simulink model "PMSM_control"  (R2021a)
settings: Solver=ode4  StartTime=0.0  StopTime=1  FixedStep=1e-5  RelTol=1e-3
libraries: spsMosfetLib x6, spsCurrentMeasurementLib x3, spsDCVoltageSourceLib x1, pid_lib x1, spsPermanentMagnetSynchronousMachineLib x1, spspowerguiLib x1
settings Model: Creator=322-PC  LastModifiedBy=juhyung
settings SolverCC: AlgebraicLoopSolver=TrustRegion
settings OptimizationCC: LifeSpan=inf
settings DebuggingCC: SFMachineParentedDataDiag=warning  ArithmeticOperatorsInVariantConditions=warning
settings SFSimCC: CustomCodeUndefinedFunction=UseInterfaceOnly
settings CodeAppCC: StateflowObjectComments=on

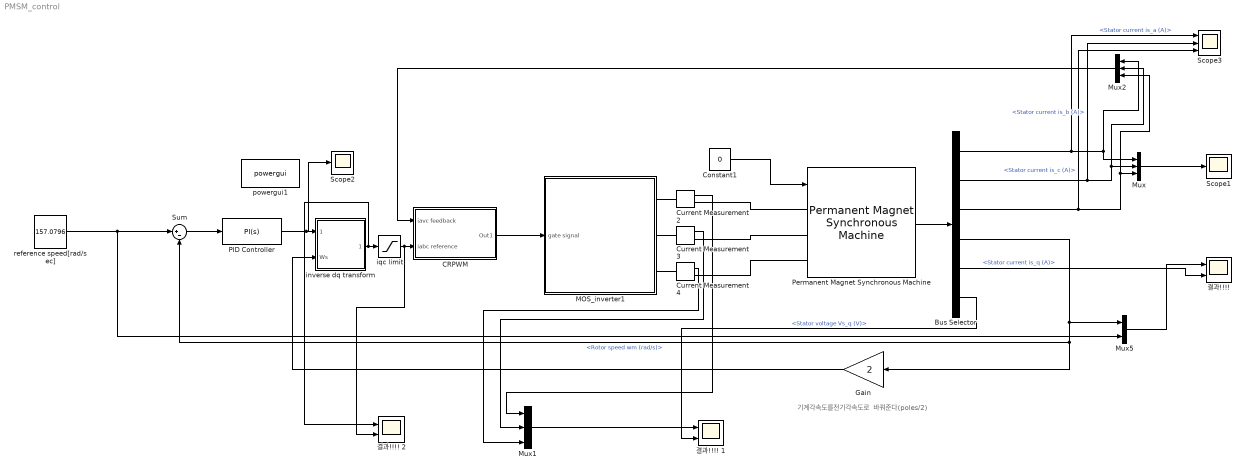
== system PMSM_control ==
  note: 기계각속도를전기각속도로 바꿔준다(poles/2)
  Bus Selector : BusSelector  OutputSignals=Stator current is_a (A),Stator current is_b (A),Stator current is_c (A),Rotor speed wm (rad/s),Stator current is_q (A),Stator voltage Vs_q (V)
  "CRPWM " : Subsystem
  Constant1 : Constant  Value=0
  Current Measurement2 : spsCurrentMeasurementLib/Current Measurement  PhasorSimulation=off  OutputType=Complex  PSBequivalent=0
  Current Measurement3 : spsCurrentMeasurementLib/Current Measurement  PhasorSimulation=off  OutputType=Complex  PSBequivalent=0
  Current Measurement4 : spsCurrentMeasurementLib/Current Measurement  PhasorSimulation=off  OutputType=Complex  PSBequivalent=0
  Gain : Gain  Gain=2
  MOS_inverter1 : Subsystem
  Mux : Mux  Inputs=3
  Mux1 : Mux  Inputs=3
  Mux2 : Mux  Inputs=3
  Mux5 : Mux  Inputs=2
  PID Controller : pid_lib/PID Controller  Controller=PI  Form=Parallel  TimeDomain=Continuous-time  UseExternalTs=off  SampleTime=-1  IntegratorMethod=Forward Euler  FilterMethod=Forward Euler  ControllerParametersSource=internal  P=0.00055  I=0.00303  D=0  UseFilter=on  N=100  TunerSelectOption=Transfer Function Based (PID Tuner App)  InitialConditionSource=internal  InitialConditionForIntegrator=0  InitialConditionForFilter=0  DifferentiatorICPrevScaledInput=0  ExternalReset=none  TrackingMode=off  Kt=1  LimitOutput=off  SatLimitsSource=internal  UpperSaturationLimit=inf  LowerSaturationLimit=-inf  LinearizeAsGain=on  AntiWindupMode=none  Kb=1  POutMin=[]  POutMax=[]  IOutMin=[]  IOutMax=[]  DOutMin=[]  DOutMax=[]  NOutMin=[]  NOutMax=[]  SumOutMin=[]  SumOutMax=[]  SaturationOutMin=[]  SaturationOutMax=[]  PParamMin=[]  PParamMax=[]  IParamMin=[]  IParamMax=[]  DParamMin=[]  DParamMax=[]  NParamMin=[]  NParamMax=[]  KbParamMin=[]  KbParamMax=[]  KtParamMin=[]  KtParamMax=[]  KbOutMin=[]  KbOutMax=[]  KtOutMin=[]  KtOutMax=[]  IntegratorOutMin=[]  IntegratorOutMax=[]  FilterOutMin=[]  FilterOutMax=[]  SumI1OutMin=[]  SumI1OutMax=[]  SumI2OutMin=[]  SumI2OutMax=[]  SumI3OutMin=[]  SumI3OutMax=[]  SumI4OutMin=[]  SumI4OutMax=[]  SumDOutMin=[]  SumDOutMax=[]  DifferentiatorOutMin=[]  DifferentiatorOutMax=[]  FilterDiffOutCoefMin=[]  FilterDiffOutCoefMax=[]  ReciprocalOutMin=[]  ReciprocalOutMax=[]  SumDenOutMin=[]  SumDenOutMax=[]  SumNumOutMin=[]  SumNumOutMax=[]  DivideOutMin=[]  DivideOutMax=[]  UdiffTsProdOutMin=[]  UdiffTsProdOutMax=[]  NTsProdOutMin=[]  NTsProdOutMax=[]  UintegralTsProdOutMin=[]  UintegralTsProdOutMax=[]  UngainTsProdOutMin=[]  UngainTsProdOutMax=[]  IntegratorContinuousStateAttributes=''  IntegratorStateMustResolveToSignalObject=off  IntegratorRTWStateStorageClass=Auto  FilterContinuousStateAttributes=''  FilterStateMustResolveToSignalObject=off  FilterRTWStateStorageClass=Auto  ParallelPVariant=InternalParameters  IdealPVariant=Disabled  IVariant=InternalParameters  DVariant=Disabled  IntegratorVariant=Continuous  SatVariant=Disabled  AWVariant=Passthrough  PCopyVariant=Disabled  TRVariant=Disabled  FdbkBlocksVariant=Forward  IdealPFdbkVariant=Disabled  SatFdbkVariant=Disabled  DerivativeFilterVariant=Disabled  NVariant=Disabled  NCopyVariant=Disabled_SignalSpec  FilterICVariant=Disabled  IntegratorICVariant=InternalICs  ExternalResetVariant=Disabled  TRSumVariant=Passthrough  SumFdbkVariant=Disabled  SumVariant=Sum_PI  TsampFilterVariant=InternalTs  TsampNgainVariant=Passthrough  TsampIntegralVariant=Passthrough  ExternalSaturationOutDataTypeStr=Inherit: Same as second input
  Permanent Magnet Synchronous Machine : spsPermanentMagnetSynchronousMachineLib/Permanent Magnet Synchronous Machine  NbPhases=3  FluxDistribution=Sinusoidal  RotorType=Round  MechanicalLoad=Torque Tm  PresetModel="01:  0.8 Nm 300 Vdc 3000 RPM - 0.8 Nm"  ShowDetailedParameters=on  MeasurementBus=off  Resistance=18.7  Inductance=8.5e-3  dqInductances=[8.5e-3,8.5e-3]  La=0.02682  MachineConstant=Flux linkage established by magnets (V.s)  Flux=0.1716  VoltageCst=62.2496  TorqueCst=0.5148  Flat=120  Mechanical=[2.26e-05 1.349e-05 2 0]  PolePairs=2  InitialConditions=[0,0, 0,0]  InitialConditions5ph=[0 0 0 0 0 0]  RefAngle=90 degrees behind phase A axis (modified Park)  IterativeDiscreteModel=Trapezoidal non iterative  TsBlock=-1  TsPowergui=0
  Scope1 : Scope
  Scope2 : Scope
  Scope3 : Scope  NumInputPorts=3
  Sum : Sum  Inputs=|+-
  inverse dq transform : Subsystem
  "iqc limit " : Saturate  UpperLimit=10  LowerLimit=-10
  powergui1 : spspowerguiLib/powergui  Priority=1  SimulationMode=Continuous  SampleTime=50e-6  frequency=60  Iterations=50  frequencyindice=0  Pbase=100e6  ErrMax=1e-4  UnitsV=kV  UnitsW=MW  buscounter=0  FunctionMessages=off  echomessages=off  EnableUseOfTLC=off  CurrentSourceSwitches=off  DisableSnubberDevices=off  DisableRonSwitches=off  DisableVfSwitches=off  DisplayEquations=off  AutomaticDiscreteSolvers=off  SolverType=Tustin/Backward Euler (TBE)  Interpol=off  ExternalGateDelay=off  methode=off  Ts=100  x0status=blocks  SPID=on  SwTol=0  HookPort=off  NonlinearTolerance=0  nMaxIteration=15  ContinueOnMaxIteration=off  RestoreLinks=warning  ResistiveCurrentMeasurement=off  Frange=[0:2:500]  Ylog=off  Xlog=on  ShowGrid=off  save=off  variable=ZData  structure=0  ZoomFFT=off  StartTime=0.0  cycles=1  DisplayStyle=1  fundamental=60  FreqAxis=off  MaxFrequency=1000  frequencyindicesteady=1  RmsSteady=1  display=off
  "reference speed[rad/sec] " : Constant  Value=157.0796
  "결과!!!! " : Scope  NumInputPorts=2
  결과!!!! 1 : Scope  NumInputPorts=2
  결과!!!! 2 : Scope  NumInputPorts=2
  wires:
  Permanent Magnet Synchronous Machine/1 -> Bus Selector/1
  Bus Selector/1 -> Scope3/1, Mux2/1, Mux/1  "<Stator current is_a (A)>"
  Bus Selector/2 -> Scope3/2, Mux2/2, Mux/2  "<Stator current is_b (A)>"
  Bus Selector/3 -> Scope3/3, Mux2/3, Mux/3  "<Stator current is_c (A)>"
  Bus Selector/5 -> "결과!!!! "/2  "<Stator current is_q (A)>"
  Bus Selector/4 -> Gain/1, Sum/2, Mux5/1  "<Rotor speed wm (rad/s)>"
  Mux/1 -> Scope1/1
  Constant1/1 -> Permanent Magnet Synchronous Machine/1
  "CRPWM "/1(Out1) -> MOS_inverter1/1(gate signal)
  Mux2/1 -> "CRPWM "/1("iavc feedback ")
  Gain/1 -> inverse dq transform/2(Ws)
  "reference speed[rad/sec] "/1 -> Mux5/2, Sum/1
  Sum/1 -> PID Controller/1
  PID Controller/1 -> Scope2/1, inverse dq transform/1(iq_refernce)
  Mux5/1 -> "결과!!!! "/1
  inverse dq transform/1(Iabc reference) -> 결과!!!! 2/1, "iqc limit "/1
  "iqc limit "/1 -> 결과!!!! 2/2, "CRPWM "/2("iabc reference ")
  Current Measurement2/1 -> Mux1/1
  Current Measurement3/1 -> Mux1/2
  Current Measurement4/1 -> Mux1/3
  Mux1/1 -> 결과!!!! 1/1
  Bus Selector/6 -> 결과!!!! 1/2  "<Stator voltage Vs_q (V)>"
  connections:
  MOS_inverter1/RConn1 -- Current Measurement2/LConn1
  Current Measurement2/RConn1 -- Permanent Magnet Synchronous Machine/LConn1
  Current Measurement3/LConn1 -- MOS_inverter1/RConn2
  Current Measurement3/RConn1 -- Permanent Magnet Synchronous Machine/LConn2
  MOS_inverter1/RConn3 -- Current Measurement4/LConn1
  Current Measurement4/RConn1 -- Permanent Magnet Synchronous Machine/LConn3

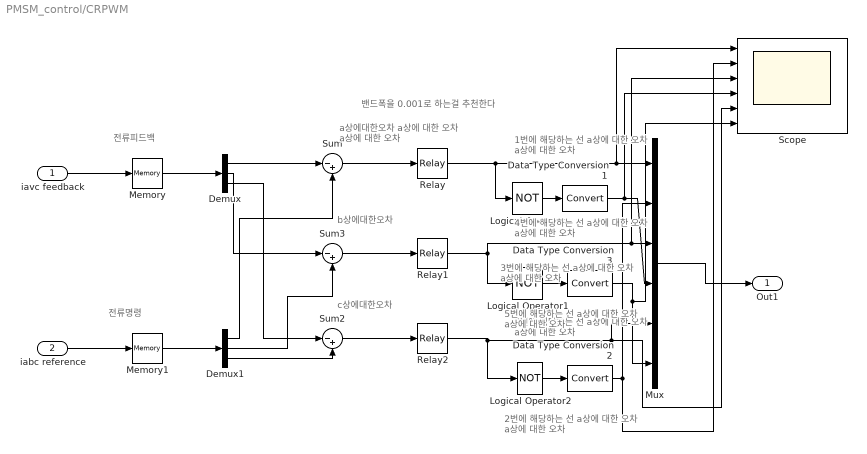
== system PMSM_control/CRPWM  ==
  note: 밴드폭을 0.001로 하는걸 추천한다
  note: 전류피드백
  note: b상에대한오차
  note: a상에대한오차
      | a상에 대한 오차
      | a상에 대한 오차
  note: c상에대한오차
  note: 1번에 해당하는 선
      | a상에 대한 오차
      | a상에 대한 오차
  note: 4번에 해당하는 선
      | a상에 대한 오차
      | a상에 대한 오차
  note: 3번에 해당하는 선
      | a상에 대한 오차
      | a상에 대한 오차
  note: 6번에 해당하는 선
      | a상에 대한 오차
      | a상에 대한 오차
  note: 5번에 해당하는 선
      | a상에 대한 오차
      | a상에 대한 오차
  note: 2번에 해당하는 선
      | a상에 대한 오차
      | a상에 대한 오차
  note: 전류명령
  "iavc feedback " : Inport
  "iabc reference " : Inport  Port=2
  Data Type Conversion1 : DataTypeConversion
  Data Type Conversion2 : DataTypeConversion
  Data Type Conversion3 : DataTypeConversion
  Demux : Demux  Outputs=3
  Demux1 : Demux  Outputs=3
  Logical Operator : Logic  Operator=NOT  AllPortsSameDT=off
  Logical Operator1 : Logic  Operator=NOT  AllPortsSameDT=off
  Logical Operator2 : Logic  Operator=NOT  AllPortsSameDT=off
  Memory : Memory
  Memory1 : Memory
  Mux : Mux  Inputs=6
  Relay : Relay  OnSwitchValue=1e-4  OffSwitchValue=-1e-4
  Relay1 : Relay  OnSwitchValue=1e-4  OffSwitchValue=-1e-4
  Relay2 : Relay  OnSwitchValue=1e-4  OffSwitchValue=-1e-4
  Scope : Scope  NumInputPorts=6
  Sum : Sum  Inputs=|-+
  Sum2 : Sum  Inputs=|-+
  Sum3 : Sum  Inputs=|-+
  Out1 : Outport  VectorParamsAs1DForOutWhenUnconnected=off
  wires:
  Relay2/1 -> Scope/5, Mux/5, Logical Operator2/1
  Logical Operator2/1 -> Data Type Conversion2/1
  "iavc feedback "/1 -> Memory/1
  Sum/1 -> Relay/1
  Relay1/1 -> Logical Operator1/1, Scope/3, Mux/3
  Demux/2 -> Sum3/1
  Data Type Conversion1/1 -> Scope/4, Mux/4
  Relay/1 -> Scope/1, Mux/1, Logical Operator/1
  Demux/3 -> Sum2/1
  Memory/1 -> Demux/1
  Memory1/1 -> Demux1/1
  Logical Operator/1 -> Data Type Conversion1/1
  Demux1/1 -> Sum/2
  Sum3/1 -> Relay1/1
  Demux1/3 -> Sum2/2
  Sum2/1 -> Relay2/1
  Demux1/2 -> Sum3/2
  Demux/1 -> Sum/1
  Logical Operator1/1 -> Data Type Conversion3/1
  Mux/1 -> Out1/1
  "iabc reference "/1 -> Memory1/1
  Data Type Conversion3/1 -> Scope/6, Mux/6
  Data Type Conversion2/1 -> Mux/2, Scope/2

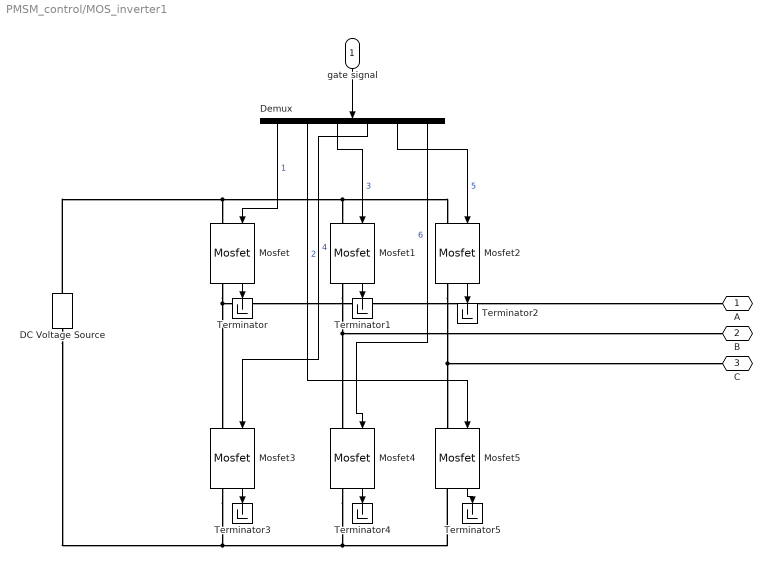
== system PMSM_control/MOS_inverter1 ==
  gate signal : Inport
  DC Voltage Source : spsDCVoltageSourceLib/DC Voltage Source  Amplitude=300  Measurements=None
  Demux : Demux  Outputs=6
  Mosfet{,1..5} (6 alike) : spsMosfetLib/Mosfet  Ron=0.1  Lon=0  Rd=0.01  Vfd=0  IC=0  Rs=1e5  Cs=inf  Measurements=on
  Terminator{,1..5} (6 alike) : Terminator
  A : PMIOPort  Side=Right
  B : PMIOPort  Port=2  Side=Right
  C : PMIOPort  Port=3  Side=Right
  wires:
  Mosfet4/1 -> Terminator4/1
  Mosfet1/1 -> Terminator1/1
  Mosfet/1 -> Terminator/1
  Mosfet3/1 -> Terminator3/1
  Mosfet5/1 -> Terminator5/1
  Demux/6 -> Mosfet4/1  "6"
  Mosfet2/1 -> Terminator2/1
  Demux/1 -> Mosfet/1  "1"
  Demux/3 -> Mosfet1/1  "3"
  Demux/5 -> Mosfet2/1  "5"
  Demux/2 -> Mosfet5/1  "2"
  Demux/4 -> Mosfet3/1  "4"
  gate signal/1 -> Demux/1
  connections:
  DC Voltage Source/RConn1 -- Mosfet1/LConn1 -- Mosfet2/LConn1 -- Mosfet/LConn1
  Mosfet/RConn1 -- Mosfet3/LConn1 -- A/RConn1
  Mosfet1/RConn1 -- Mosfet4/LConn1 -- B/RConn1
  Mosfet2/RConn1 -- C/RConn1 -- Mosfet5/LConn1
  DC Voltage Source/LConn1 -- Mosfet5/RConn1 -- Mosfet4/RConn1 -- Mosfet3/RConn1

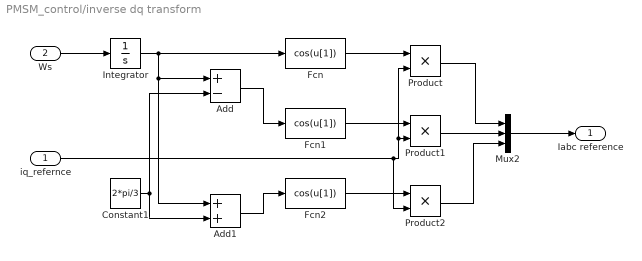
== system PMSM_control/inverse dq transform ==
  iq_refernce : Inport
  Ws : Inport  Port=2
  Add : Sum  Inputs=+-
  Add1 : Sum
  Constant1 : Constant  Value=2*pi/3
  Fcn : Fcn  Expr=cos(u[1])
  Fcn1 : Fcn  Expr=cos(u[1])
  Fcn2 : Fcn  Expr=cos(u[1])
  Integrator : Integrator
  Mux2 : Mux  Inputs=3
  Product : Product
  Product1 : Product
  Product2 : Product
  Iabc reference : Outport  VectorParamsAs1DForOutWhenUnconnected=off
  wires:
  Product/1 -> Mux2/1
  Constant1/1 -> Add/2, Add1/2
  iq_refernce/1 -> Product2/2, Product1/2, Product/2
  Integrator/1 -> Add1/1, Add/1, Fcn/1
  Add/1 -> Fcn1/1
  Add1/1 -> Fcn2/1
  Product1/1 -> Mux2/2
  Fcn2/1 -> Product2/1
  Fcn/1 -> Product/1
  Fcn1/1 -> Product1/1
  Product2/1 -> Mux2/3
  Ws/1 -> Integrator/1
  Mux2/1 -> Iabc reference/1
